simulink model "sampleModel1400_4"  (R2023a)
settings: Solver=VariableStepAuto  StartTime=0.0  StopTime=10.0  RelTol=1e-3
libraries: hdlsllib x5, simulink x1
settings Model: Creator=user1  LastModifiedBy=user1

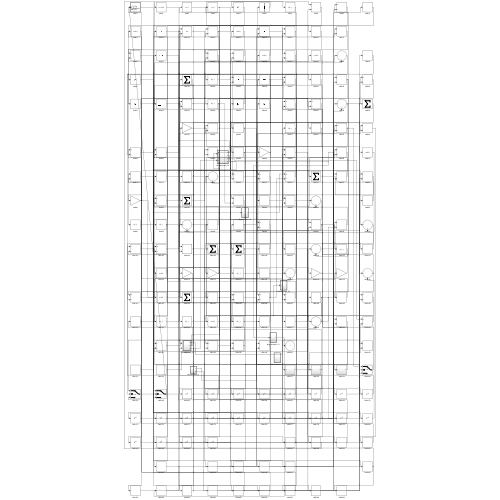
[thumbnail: Simulink's stored preview of the top-level diagram]
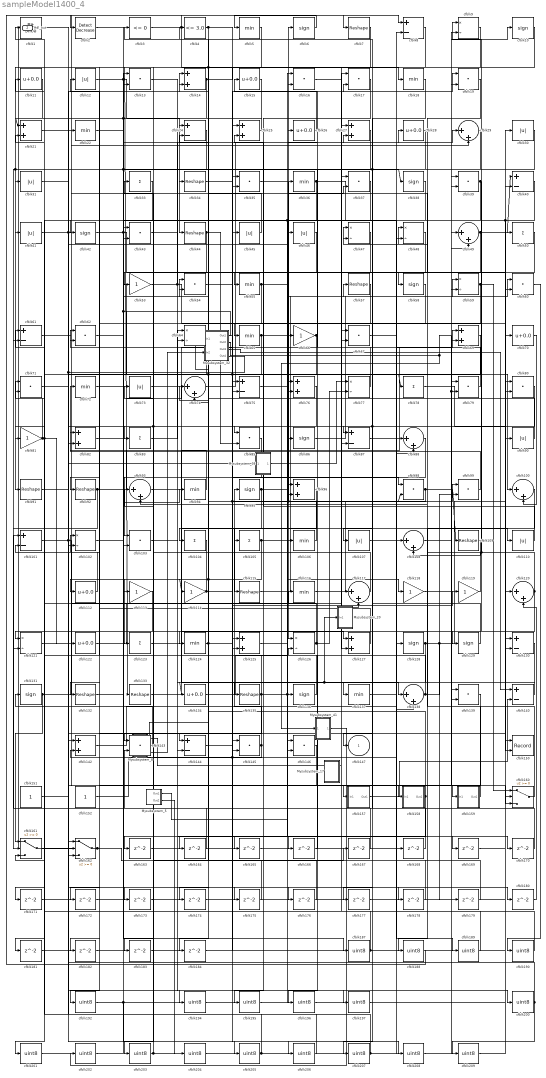
== system sampleModel1400_4 ==
  Mysubsystem_17 : Subsystem  TreatAsAtomicUnit=on  RTWFcnName=Mysubsystem_17
      settings: RTWFcnNameOpts=User specified  RTWFileNameOpts=Use function name
  Mysubsystem_20 : Subsystem  TreatAsAtomicUnit=on  RTWFcnName=Mysubsystem_20
      settings: RTWFcnNameOpts=User specified  RTWFileNameOpts=Use function name
  Mysubsystem_32 : Subsystem  TreatAsAtomicUnit=on  RTWFcnName=Mysubsystem_32
      settings: RTWFcnNameOpts=User specified  RTWFileNameOpts=Use function name
  Mysubsystem_36 : Subsystem  TreatAsAtomicUnit=on  RTWFcnName=Mysubsystem_36
      settings: RTWFcnNameOpts=User specified  RTWFileNameOpts=Use function name
  Mysubsystem_41 : Subsystem  TreatAsAtomicUnit=on  RTWFcnName=Mysubsystem_41
      settings: RTWFcnNameOpts=User specified  RTWFileNameOpts=Use function name
  Mysubsystem_5 : Subsystem  TreatAsAtomicUnit=on  RTWFcnName=Mysubsystem_5
      settings: RTWFcnNameOpts=User specified  RTWFileNameOpts=Use function name
  Mysubsystem_8 : Subsystem  TreatAsAtomicUnit=on  RTWFcnName=Mysubsystem_8
      settings: RTWFcnNameOpts=User specified  RTWFileNameOpts=Use function name
  cfblk1 : hdlsllib/Logic and Bit Operations/Bit Slice  lidx=7  ridx=0
  cfblk{6,10,38,42,58,86,95,128..129,131,136} (11 alike) : Signum
  cfblk{29,49,74,88,93,100,108,117,120,138} (10 alike) : Sum  Inputs=|++  OutDataTypeStr=uint8
  cfblk{8,24,40,61,75,87,101,130,140,144} (10 alike) : Sum  Inputs=+-  OutDataTypeStr=uint8
  cfblk{9,47..48,59,64,77,102,121,126} (9 alike) : Product  Inputs=*/  OutDataTypeStr=uint8  RndMeth=Zero  SaturateOnIntegerOverflow=on
  cfblk{13,16..17,19,35,37,39,43,54,60,62,67,71,79..80,85,98..99,103,139,143,145..146} (23 alike) : DotProduct  OutDataTypeStr=uint8
  cfblk{33,50,78,83,104..105,123} (7 alike) : Sum  Inputs=+  OutDataTypeStr=uint8
  cfblk{5,18,22,36,55,65,72,94,106,116,124,137} (12 alike) : MinMax  OutDataTypeStr=uint8
  cfblk{12,30..31,41,45..46,73,90,107,110} (10 alike) : Abs  OutDataTypeStr=uint8  SaturateOnIntegerOverflow=off
  cfblk{7,34,44,57,91..92,109,115,132..133,135} (11 alike) : Reshape
  cfblk{11,15,26,28,70,112,122,134} (8 alike) : Bias  Bias=0.0  SaturateOnIntegerOverflow=off
  cfblk{53,66,81,113..114,118..119} (7 alike) : Gain  OutDataTypeStr=uint8
  cfblk{14,21,25,27,69,76,82,96,125,127,142} (11 alike) : Sum  OutDataTypeStr=uint8
  cfblk150 : Record  FileSettingsInternal="{\"entries\":[{\"content\":{\"excelSettings\":{\"content\":{},\"type\":\"Streamout.ExcelSettings\"}},\"type\":\"Streamout.FileSettingStorage\",\"uuid\":\"\"}],\"packageUris\":[\"http:\\/\\/schema.mathworks.com\\/mf0\\/streamout_blocks\\/R2020a\"],\"version\":\"1.0\"}"  Layout=[1 1]  SignalsInternal="{\"entries\":[{\"content\":{\"signals\":[{\"content\":{\"blockPath\":[],\"dimensions\":[1],\"domain\":\"\",\"lineColor\":\"#a2142f\",\"plots\":[1],\"port\":1,\"signalID\":10637,\"signalName\":\"cfblk53\"},\"type\":\"RecordBlkView.Signal\",\"uuid\":\"\"},{\"content\":{\"blockPath\":[],\"dimensions\":[1],\"domain\":\"\",\"lineColor\":\"#139fff\",\"plots\":[1],\"port\":2,\"signalID\":10640,\"signalName\":\"cfblk52\"},\"type\":\"RecordBlkView.Signal\",\"uuid\":\"\"}]},\"type\":\"RecordBlkView.InputSignals\",\"uuid\":\"\"}],\"packageUris\":[\"http:\\/\\/schema.mathworks.com\\/mf0\\/streamout_blocks\\/R2020a\"],\"version\":\"1.0\"}"  VisualizationBindings="{\"xyplotplugin\":{\"info\":[{\"series\":[{\"bindingParametersList\":[{\"parameter\":\"X-Axis\",\"signalID\":10637,\"signalName\":\"cfblk53\"},{\"parameter\":\"Y-Axis\",\"signalID\":10640,\"signalName\":\"cfblk52\"}],\"seriesID\":21453}],\"subplotID\":1}]}}"  CompatibilityTag=XY  st=-1
  cfblk151 : Constant  OutDataTypeStr=uint8  SampleTime=-1
  cfblk152 : Constant  OutDataTypeStr=uint8  SampleTime=-1
  cfblk157 : Subsystem
      settings: LibrarySourceBlock=|
      | hdlsllib/Ports &
      | Subsystems/Subsystem
  cfblk158 : Subsystem
      settings: LibrarySourceBlock=|
      | hdlsllib/Ports &
      | Subsystems/Subsystem
  cfblk159 : Subsystem
      settings: LibrarySourceBlock=|
      | hdlsllib/Ports &
      | Subsystems/Subsystem
  cfblk160 : Switch  OutDataTypeStr=uint8  SaturateOnIntegerOverflow=off  InputSameDT=off
  cfblk161 : Switch  OutDataTypeStr=uint8  SaturateOnIntegerOverflow=off  InputSameDT=off
  cfblk162 : Switch  OutDataTypeStr=uint8  SaturateOnIntegerOverflow=off  InputSameDT=off
  cfblk{163..184} (22 alike) : Delay  SampleTime=1
  cfblk{187..190,192,194..197,200..209} (19 alike) : DataTypeConversion  OutDataTypeStr=uint8  SaturateOnIntegerOverflow=off  RndMeth=Floor
  cfblk2 : simulink/Logic and Bit Operations/Detect Decrease  vinit=0.0  OutDataTypeStr=uint8
      settings: LibrarySourceBlock=|
      | hdlsllib/Logic and Bit
      | Operations/Detect
      | Decrease
  cfblk3 : hdlsllib/Logic and Bit Operations/Compare To Zero  relop=<=  OutDataTypeStr=uint8
  cfblk4 : hdlsllib/Logic and Bit Operations/Compare To Constant  relop=<=  const=3.0  OutDataTypeStr=uint8
  cfblk147 : Outport  OutDataTypeStr=uint8  VectorParamsAs1DForOutWhenUnconnected=off
  Hdl_out : Outport  Port=2  OutDataTypeStr=uint8
  wires:
  cfblk5/1 -> cfblk133/1, cfblk34/1
  cfblk47/1 -> cfblk126/1
  cfblk131/1 -> cfblk7/1, cfblk161/1
  cfblk94/1 -> cfblk72/1
  cfblk129/1 -> cfblk3/1
  cfblk88/1 -> cfblk103/1
  cfblk102/1 -> cfblk28/1
  cfblk120/1 -> cfblk47/1, cfblk9/1, cfblk181/1
  cfblk74/1 -> cfblk29/1
  cfblk86/1 -> cfblk59/1
  cfblk145/1 -> cfblk95/1, cfblk142/2
  cfblk138/1 -> cfblk12/1, cfblk99/2
  cfblk116/1 -> cfblk99/1
  cfblk115/1 -> cfblk60/1
  cfblk128/1 -> cfblk30/1, cfblk179/1, cfblk144/2
  cfblk93/1 -> cfblk110/1
  cfblk157/1(Out1) -> cfblk140/2
  cfblk123/1 -> cfblk127/1
  cfblk117/1 -> cfblk73/1
  cfblk106/1 -> cfblk6/1, cfblk4/1
  cfblk35/1 -> cfblk86/1
  cfblk98/1 -> cfblk109/1, cfblk96/2
  cfblk11/1 -> cfblk91/1
  cfblk55/1 -> cfblk65/1, cfblk160/2
  cfblk28/1 -> cfblk87/1, cfblk162/2
  cfblk29/1 -> cfblk41/1, cfblk121/2
  cfblk101/1 -> cfblk157/1(In1), cfblk159/1(In1), cfblk46/1
  cfblk30/1 -> cfblk92/1
  cfblk3/1 -> cfblk8/1, cfblk27/1
  cfblk70/1 -> cfblk100/2
  cfblk73/1 -> cfblk137/1
  cfblk134/1 -> cfblk106/1
  cfblk99/1 -> cfblk82/1
  cfblk39/1 -> cfblk147/1, cfblk129/1
  cfblk48/1 -> cfblk125/2
  cfblk58/1 -> cfblk127/2
  cfblk61/1 -> cfblk29/2
  cfblk10/1 -> cfblk31/1
  cfblk135/1 -> cfblk17/2, cfblk158/1(In1), cfblk62/1, cfblk182/1
  cfblk114/1 -> cfblk112/1, cfblk197/1
  cfblk133/1 -> cfblk49/1
  cfblk40/1 -> cfblk81/1, cfblk76/2, cfblk60/2
  cfblk151/1 -> cfblk22/1
  cfblk8/1 -> cfblk53/1
  cfblk104/1 -> cfblk132/1
  cfblk82/1 -> cfblk43/1
  cfblk144/1 -> cfblk45/1, cfblk98/2
  cfblk59/1 -> cfblk160/1, cfblk172/1
  cfblk19/1 -> cfblk58/1
  cfblk108/1 -> cfblk10/1
  cfblk26/1 -> cfblk15/1
  cfblk49/1 -> cfblk40/1, cfblk145/2
  cfblk140/1 -> Mysubsystem_20/1(In1), cfblk134/1
  cfblk112/1 -> cfblk61/1
  cfblk36/1 -> cfblk88/1, cfblk74/2
  cfblk95/1 -> cfblk115/1, cfblk57/1
  cfblk125/1 -> cfblk138/1
  cfblk142/1 -> cfblk69/1
  cfblk83/1 -> cfblk64/1
  cfblk53/1 -> cfblk150/1, cfblk27/2
  cfblk130/1 -> cfblk207/1
  cfblk124/1 -> cfblk119/1, cfblk144/1
  cfblk72/1 -> cfblk37/2
  cfblk122/1 -> cfblk116/1
  cfblk16/1 -> cfblk117/2
  cfblk92/1 -> cfblk35/1, cfblk161/2
  cfblk24/1 -> cfblk61/2
  cfblk110/1 -> cfblk25/2
  cfblk12/1 -> cfblk44/1, cfblk76/1
  cfblk152/1 -> cfblk108/1, cfblk35/2
  cfblk132/1 -> cfblk94/1
  cfblk159/1(Out1) -> cfblk36/1
  cfblk22/1 -> cfblk38/1, cfblk48/2
  cfblk80/1 -> cfblk105/1, cfblk107/1
  cfblk160/1 -> cfblk62/2
  cfblk90/1 -> cfblk54/1
  cfblk146/1 -> cfblk192/1
  cfblk77/1 -> cfblk26/1
  cfblk1/1 -> cfblk205/1
  cfblk15/1 -> cfblk64/2
  cfblk25/1 -> cfblk24/1
  cfblk137/1 -> cfblk128/1
  cfblk121/1 -> cfblk87/2
  cfblk91/1 -> cfblk143/1
  cfblk78/1 -> cfblk120/1
  cfblk6/1 -> cfblk5/1
  cfblk34/1 -> cfblk19/1
  cfblk57/1 -> cfblk135/1
  cfblk13/1 -> cfblk200/1
  cfblk4/1 -> cfblk75/1, cfblk184/1
  cfblk65/1 -> cfblk83/1, cfblk118/1
  cfblk69/1 -> cfblk104/1, cfblk162/3
  cfblk127/1 -> cfblk102/1
  cfblk7/1 -> cfblk102/2
  cfblk81/1 -> cfblk122/1, cfblk21/2, cfblk71/1
  cfblk64/1 -> cfblk66/1, cfblk171/1
  cfblk42/1 -> cfblk70/1, cfblk180/1
  cfblk41/1 -> cfblk78/1, cfblk75/2, cfblk17/1
  cfblk79/1 -> cfblk48/1
  cfblk105/1 -> cfblk123/1, cfblk169/1
  cfblk2/1 -> cfblk187/1
  cfblk66/1 -> cfblk85/1, cfblk16/2
  cfblk75/1 -> cfblk96/1
  cfblk62/1 -> cfblk54/2
  cfblk46/1 -> cfblk55/1
  cfblk45/1 -> cfblk14/1
  cfblk37/1 -> cfblk124/1
  cfblk50/1 -> cfblk203/1
  cfblk9/1 -> cfblk42/1
  cfblk143/1 -> cfblk101/2
  cfblk38/1 -> cfblk103/2
  cfblk54/1 -> cfblk98/1
  cfblk14/1 -> cfblk43/2, cfblk21/1, cfblk18/1
  cfblk44/1 -> cfblk85/2, cfblk163/1
  cfblk118/1 -> cfblk19/2
  cfblk33/1 -> cfblk121/1
  cfblk126/1 -> cfblk71/2, cfblk77/2
  cfblk119/1 -> cfblk93/2
  cfblk158/1(Out1) -> cfblk74/1, cfblk183/1
  cfblk136/1 -> cfblk11/1
  cfblk109/1 -> cfblk108/2
  cfblk76/1 -> cfblk113/1, cfblk82/2
  cfblk163/1 -> cfblk138/2
  cfblk85/1 -> cfblk164/1
  cfblk164/1 -> cfblk101/1
  cfblk17/1 -> cfblk165/1
  cfblk165/1 -> cfblk37/1
  cfblk103/1 -> cfblk166/1
  cfblk166/1 -> cfblk126/2
  cfblk162/1 -> cfblk167/1, Hdl_out/1
  cfblk167/1 -> cfblk143/2
  cfblk87/1 -> cfblk168/1
  cfblk168/1 -> cfblk47/2
  cfblk169/1 -> cfblk80/2
  cfblk107/1 -> cfblk170/1
  cfblk170/1 -> cfblk25/1
  cfblk171/1 -> cfblk40/2
  cfblk172/1 -> cfblk49/2
  cfblk31/1 -> cfblk173/1
  cfblk173/1 -> cfblk59/2
  cfblk96/1 -> cfblk174/1
  cfblk174/1 -> cfblk117/1
  cfblk161/1 -> cfblk175/1
  cfblk175/1 -> cfblk125/1
  cfblk43/1 -> cfblk176/1
  cfblk176/1 -> cfblk24/2
  cfblk18/1 -> cfblk177/1
  cfblk177/1 -> cfblk39/2
  cfblk21/1 -> cfblk178/1
  cfblk178/1 -> cfblk93/1
  cfblk179/1 -> cfblk16/1
  cfblk180/1 -> cfblk120/2
  cfblk181/1 -> cfblk69/2
  cfblk182/1 -> cfblk145/1
  cfblk183/1 -> cfblk8/2
  cfblk187/1 -> cfblk131/1, cfblk90/1
  cfblk100/1 -> cfblk188/1
  cfblk188/1 -> cfblk2/1
  cfblk67/1 -> cfblk189/1
  cfblk189/1 -> cfblk79/1
  cfblk60/1 -> cfblk190/1
  cfblk190/1 -> cfblk67/1
  cfblk192/1 -> cfblk80/1, cfblk208/1
  cfblk71/1 -> cfblk194/1
  cfblk194/1 -> cfblk146/2
  cfblk139/1 -> cfblk195/1
  cfblk195/1 -> cfblk136/1
  cfblk27/1 -> cfblk196/1
  cfblk196/1 -> cfblk139/1
  cfblk197/1 -> cfblk139/2
  cfblk200/1 -> cfblk142/1, cfblk209/1
  cfblk113/1 -> cfblk201/1
  cfblk201/1 -> cfblk13/1
  cfblk202/1 -> cfblk13/2
  cfblk203/1 -> cfblk79/2, cfblk9/2, cfblk33/1
  cfblk204/1 -> cfblk50/1
  cfblk205/1 -> cfblk161/3, cfblk39/1
  cfblk184/1 -> cfblk206/1
  cfblk206/1 -> cfblk1/1
  cfblk207/1 -> cfblk162/1, cfblk88/2
  cfblk208/1 -> cfblk130/1
  cfblk209/1 -> cfblk130/2
  Mysubsystem_5/1(Out1) -> cfblk146/1
  Mysubsystem_5/2(Out2) -> cfblk204/1
  Mysubsystem_8/2(Out2) -> Mysubsystem_32/1(In1), cfblk114/1
  Mysubsystem_8/1(Out1) -> cfblk67/2
  Mysubsystem_32/2(Out2) -> Mysubsystem_41/1(In1), cfblk160/3
  Mysubsystem_32/4(Out4) -> Mysubsystem_36/1(In1), cfblk14/2
  Mysubsystem_32/1(Out1) -> cfblk100/1, cfblk150/2
  Mysubsystem_8/3(y) -> Mysubsystem_32/2(In2)
  Mysubsystem_32/3(Out3) -> cfblk140/1
  Mysubsystem_36/1(Out1) -> cfblk77/1
  Mysubsystem_41/1(Out1) -> cfblk202/1

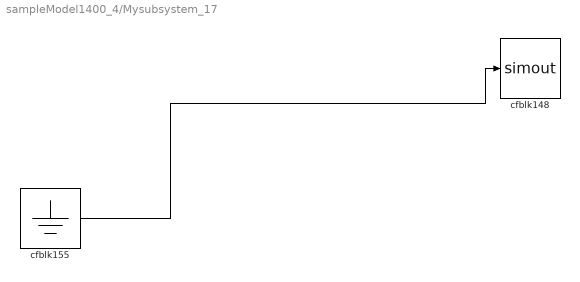
== system sampleModel1400_4/Mysubsystem_17 ==
  cfblk148 : ToWorkspace  VariableName=simout  SaveFormat=Timeseries  SampleTime=-1
  cfblk155 : Ground
  wires:
  cfblk155/1 -> cfblk148/1

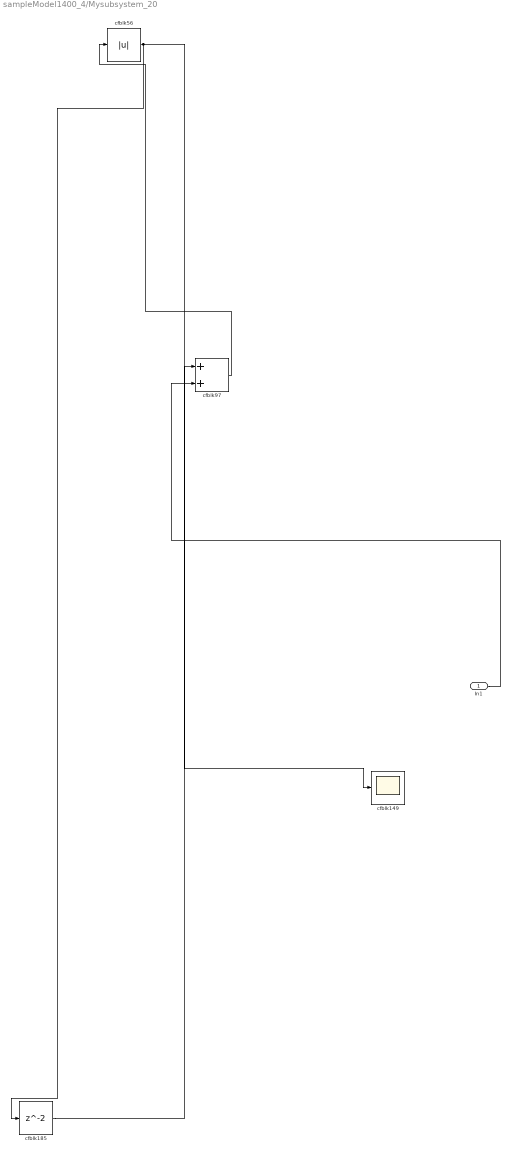
== system sampleModel1400_4/Mysubsystem_20 ==
  In1 : Inport
  cfblk149 : Scope
  cfblk185 : Delay  SampleTime=1
  cfblk56 : Abs  SaturateOnIntegerOverflow=off
  cfblk97 : Sum
  wires:
  cfblk56/1 -> cfblk149/1, cfblk185/1
  cfblk97/1 -> cfblk56/1
  cfblk185/1 -> cfblk97/1
  In1/1 -> cfblk97/2

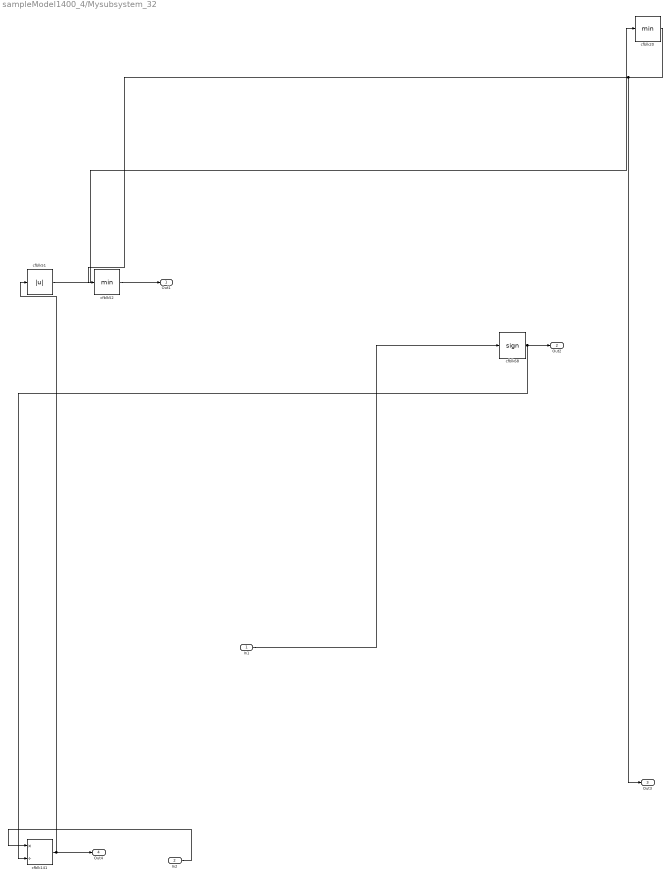
== system sampleModel1400_4/Mysubsystem_32 ==
  In1 : Inport
  In2 : Inport  Port=2
  cfblk141 : Product  Inputs=*/  RndMeth=Zero  SaturateOnIntegerOverflow=on
  cfblk20 : MinMax
  cfblk51 : Abs  SaturateOnIntegerOverflow=off
  cfblk52 : MinMax
  cfblk68 : Signum
  Out1 : Outport
  Out2 : Outport  Port=2
  Out3 : Outport  Port=3
  Out4 : Outport  Port=4
  wires:
  cfblk20/1 -> Out3/1, cfblk52/1
  cfblk68/1 -> Out2/1, cfblk141/2
  In1/1 -> cfblk68/1
  cfblk52/1 -> Out1/1
  cfblk141/1 -> Out4/1, cfblk51/1
  cfblk51/1 -> cfblk20/1
  In2/1 -> cfblk141/1

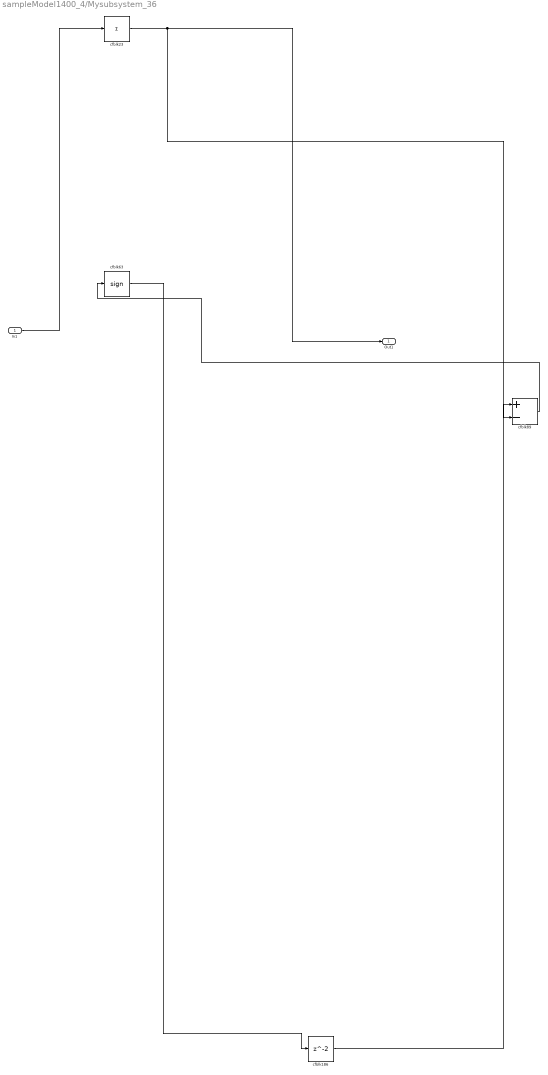
== system sampleModel1400_4/Mysubsystem_36 ==
  In1 : Inport
  cfblk186 : Delay  SampleTime=1
  cfblk23 : Sum  Inputs=+
  cfblk63 : Signum
  cfblk89 : Sum  Inputs=+-
  Out1 : Outport
  wires:
  cfblk63/1 -> cfblk186/1
  cfblk186/1 -> cfblk89/1
  cfblk89/1 -> cfblk63/1
  In1/1 -> cfblk23/1
  cfblk23/1 -> Out1/1, cfblk89/2

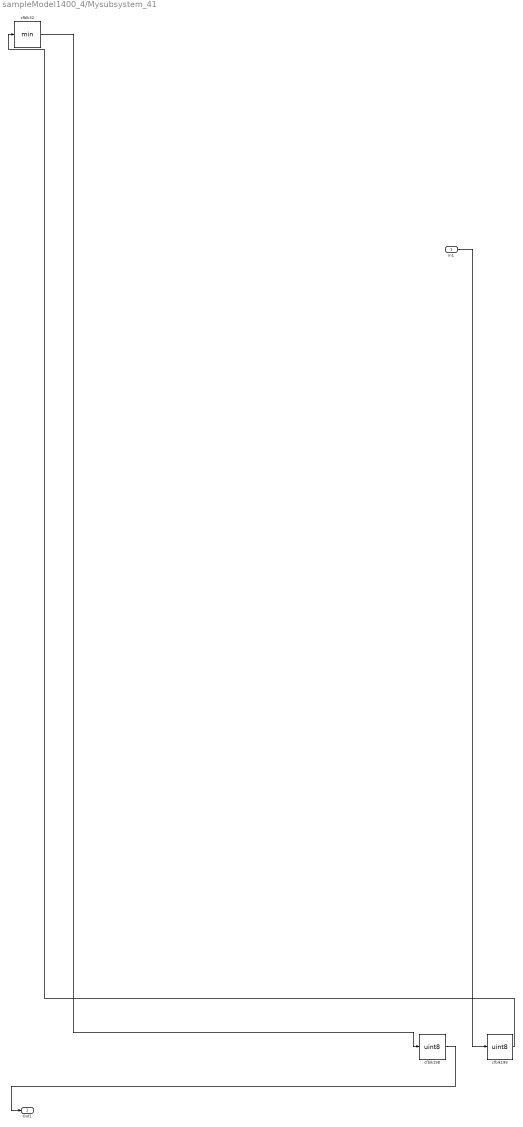
== system sampleModel1400_4/Mysubsystem_41 ==
  In1 : Inport
  cfblk198 : DataTypeConversion  OutDataTypeStr=uint8  SaturateOnIntegerOverflow=off  RndMeth=Floor
  cfblk199 : DataTypeConversion  OutDataTypeStr=uint8  SaturateOnIntegerOverflow=off  RndMeth=Floor
  cfblk32 : MinMax
  Out1 : Outport
  wires:
  cfblk32/1 -> cfblk198/1
  cfblk199/1 -> cfblk32/1
  In1/1 -> cfblk199/1
  cfblk198/1 -> Out1/1

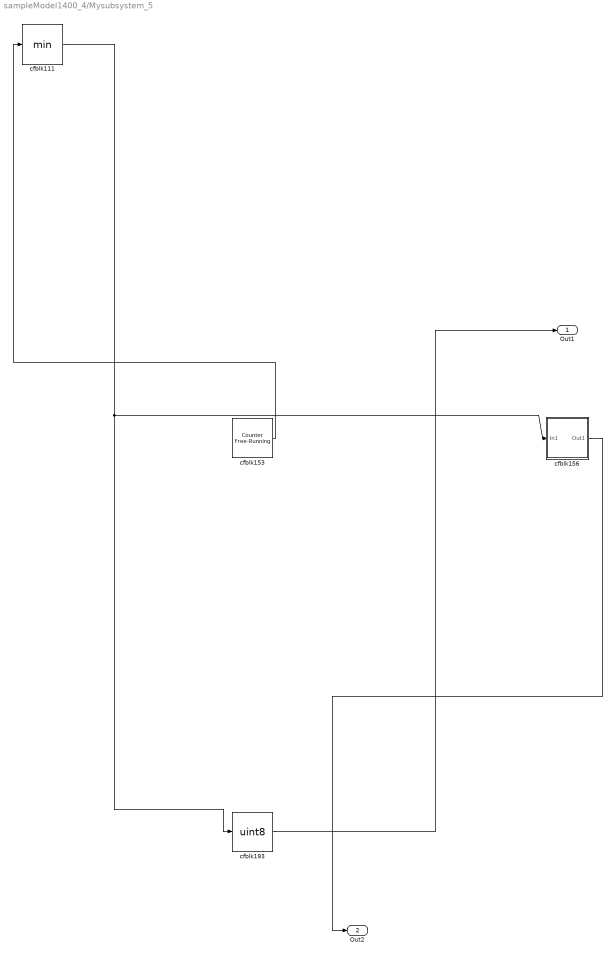
== system sampleModel1400_4/Mysubsystem_5 ==
  cfblk111 : MinMax
  cfblk153 : hdlsllib/Sources/Counter Free-Running  NumBits=16  tsamp=-1
  cfblk156 : Subsystem
      settings: LibrarySourceBlock=|
      | hdlsllib/Ports &
      | Subsystems/Subsystem
  cfblk193 : DataTypeConversion  OutDataTypeStr=uint8  SaturateOnIntegerOverflow=off  RndMeth=Floor
  Out1 : Outport
  Out2 : Outport  Port=2
  wires:
  cfblk153/1 -> cfblk111/1
  cfblk111/1 -> cfblk156/1(In1), cfblk193/1
  cfblk193/1 -> Out1/1
  cfblk156/1(Out1) -> Out2/1

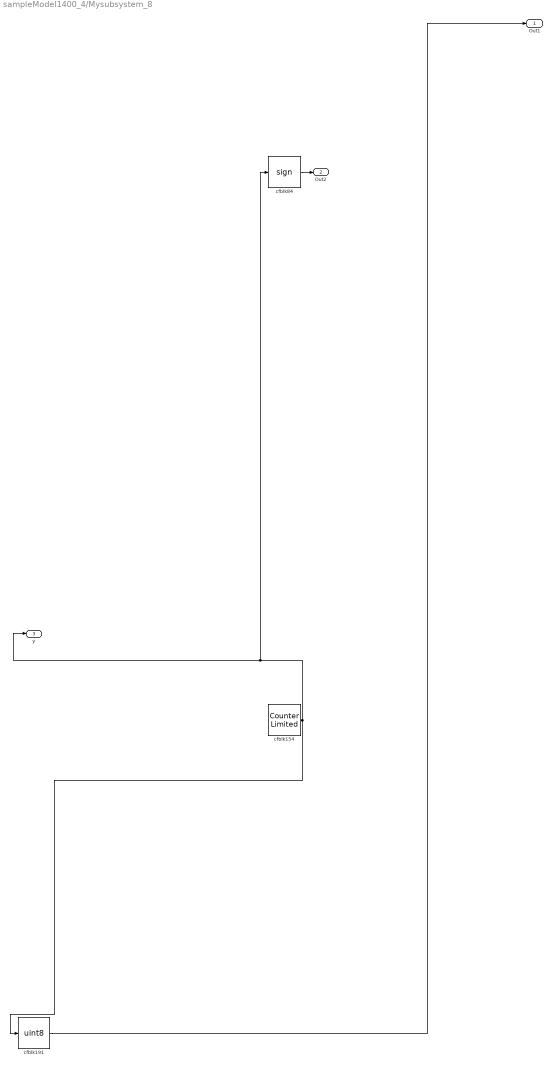
== system sampleModel1400_4/Mysubsystem_8 ==
  cfblk154 : hdlsllib/Sources/Counter Limited  uplimit=7  tsamp=-1
  cfblk191 : DataTypeConversion  OutDataTypeStr=uint8  SaturateOnIntegerOverflow=off  RndMeth=Floor
  cfblk84 : Signum
  Out1 : Outport
  Out2 : Outport  Port=2
  y : Outport  Port=3
  wires:
  cfblk154/1 -> y/1, cfblk84/1, cfblk191/1
  cfblk84/1 -> Out2/1
  cfblk191/1 -> Out1/1

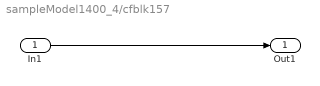
== system sampleModel1400_4/cfblk157 ==
  In1 : Inport
  Out1 : Outport
  wires:
  In1/1 -> Out1/1

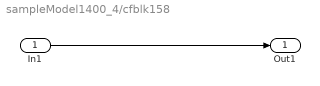
== system sampleModel1400_4/cfblk158 ==
  In1 : Inport
  Out1 : Outport
  wires:
  In1/1 -> Out1/1

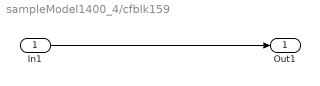
== system sampleModel1400_4/cfblk159 ==
  In1 : Inport
  Out1 : Outport
  wires:
  In1/1 -> Out1/1

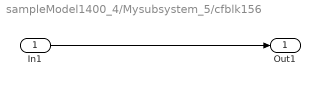
== system sampleModel1400_4/Mysubsystem_5/cfblk156 ==
  In1 : Inport
  Out1 : Outport
  wires:
  In1/1 -> Out1/1
